simulink model "CM680A_HwTq2Meas"  (R2013b)
settings: Solver=FixedStepDiscrete  SolverMode=SingleTasking  StartTime=0.0  StopTime=1  FixedStep=0.002  RelTol=1e-3
values from neighbouring files (symbols this model uses):
  ELECGLBPRM_HWTQOFFS_HWNWTMTR_F32 = DataDict.Constant    [CM680A_HwTq2Meas_DataDict.m]
  ELECGLBPRM_HWTQSATNLOWRLIM_HWNWTMTR_F32 = DataDict.Constant    [CM680A_HwTq2Meas_DataDict.m]
  ELECGLBPRM_HWTQSATNUPPRLIM_HWNWTMTR_F32 = DataDict.Constant    [CM680A_HwTq2Meas_DataDict.m]
  ELECGLBPRM_HWTQSCA_ULS_F32 = DataDict.Constant    [CM680A_HwTq2Meas_DataDict.m]
  ELECGLBPRM_NOFLT_CNT_U08 = DataDict.Constant    [CM680A_HwTq2Meas_DataDict.m]
  ELECGLBPRM_OFFSTRIMNOTPRFM_CNT_U08 = DataDict.Constant    [CM680A_HwTq2Meas_DataDict.m]
  ELECGLBPRM_PRTCLFLT_CNT_U08 = DataDict.Constant    [CM680A_HwTq2Meas_DataDict.m]
  ELECGLBPRM_SNSRINTFLT_CNT_U08 = DataDict.Constant    [CM680A_HwTq2Meas_DataDict.m]
  FLTINJ_HWTQ2MEAS_HWTQ2 = DataDict.Constant    [CM680A_HwTq2Meas_DataDict.m]
  GearIdn1 = DataDict.OpSignal    [CM680A_HwTq2Meas_DataDict.m]
  HwTq2MeasHwTq2PrtclFltFailStep = DataDict.Calibration    [CM680A_HwTq2Meas_DataDict.m]
  HwTq2MeasHwTq2PrtclFltPassStep = DataDict.Calibration    [CM680A_HwTq2Meas_DataDict.m]
undefined symbols (not defined in the file or in its folder): NtcNr1, NtcSts1, sigbuilder_block, SigQlfr1
libraries: simulink x22, NxtrNvM x3
(part 3 of 3)

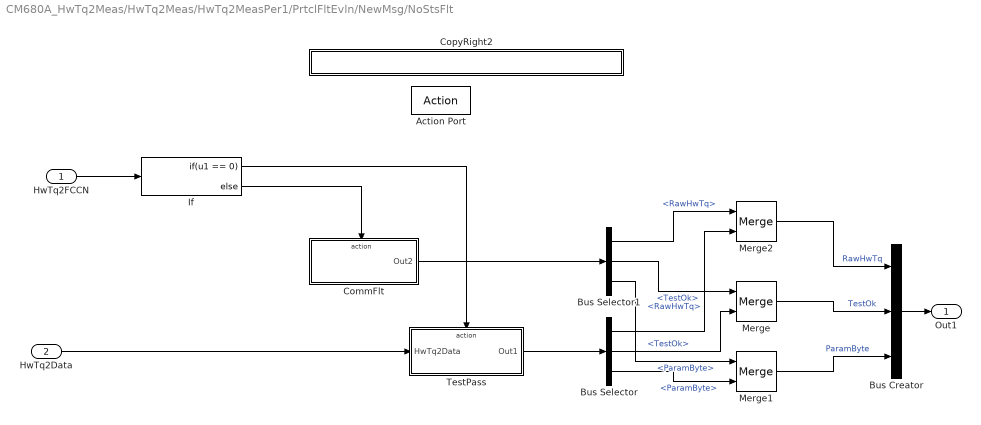
== system CM680A_HwTq2Meas/HwTq2Meas/HwTq2MeasPer1/PrtclFltEvln/NewMsg/NoStsFlt ==
  HwTq2FCCN : Inport
  HwTq2Data : Inport  Port=2
  Action Port : ActionPort  ActionType=then
  Bus Creator : BusCreator  Inputs=3
  Bus Selector : BusSelector  OutputSignals=RawHwTq,TestOk,ParamByte
  Bus Selector1 : BusSelector  OutputSignals=RawHwTq,TestOk,ParamByte
  CommFlt : Subsystem  RequirementInfo={'linktype_rmi_doors' '0000cf42 (/ESG Group/FDD Module Requirements/EA4 Specific/CM680A_HwTq2Meas)' '#CM680A_28' 'true' 'REQ: CM680A_28' '' ; 'linktype_rmi_doors' '0000cf42 (/ESG Group/FDD Module Requirements/EA4 Specific/CM680A_HwTq2Meas)' '#CM680A_48' 'true' 'REQ: CM680A_48' '' } %GIDa_a181911d_9433_49e5_ad17_4bc594fa1b0c  TreatAsAtomicUnit=on
      mask Display: disp('CommFlt')
  CopyRight2 : Subsystem  Description=|  mask(Copyright Information){none=on}
      | Copyright info block.                                               
      |                                                                     
      | Place copyright information at the top of every subsystem in design.
      mask prompts: none "No parameters"
      mask help: Place copyright information at the top of every subsystem in design.
      mask Display:
      | NxtrConf = 'Nexteer Confidential';
      | 
      | sys = bdroot; %handle for the current model ("system")
      | first = get_param(sys,'Created');
      | first = first(end-3:end);  %year is last four digits
      | 
      | last = get_param(sys,'LastModifiedDate');
      | if isempty(last)
      |     last = datestr(now,'yyyy');
      | else
      |     last = last(end-3:end);
      | end
      | 
      | if strcmp(first,last)
      |     fprintf('%s -- Copyright %s Nexteer',NxtrConf,first)
      | else
      |     fprintf('%s -- %s%s- %s Nexteer',NxtrConf,char(169),first,last)
      | end
  If : If  IfExpression=u1 == 0
  Merge : Merge
  Merge1 : Merge
  Merge2 : Merge
  TestPass : Subsystem  RequirementInfo={'linktype_rmi_doors' '0000cf42 (/ESG Group/FDD Module Requirements/EA4 Specific/CM680A_HwTq2Meas)' '#CM680A_49' 'true' 'REQ: CM680A_49' '' } %GIDa_eb2d61f5_a171_4ae7_8550_49e90430938b  TreatAsAtomicUnit=on
      mask Display: disp('TESTPASS')
  Out1 : Outport
  wires:
  HwTq2FCCN/1 -> If/1
  If/1 -> TestPass/Action
  If/2 -> CommFlt/Action
  Merge/1 -> Bus Creator/2  "TestOk"
  Merge1/1 -> Bus Creator/3  "ParamByte"
  Merge2/1 -> Bus Creator/1  "RawHwTq"
  TestPass/1(Out1) -> Bus Selector/1
  CommFlt/1(Out2) -> Bus Selector1/1
  Bus Selector1/1 -> Merge2/1  "<RawHwTq>"
  Bus Selector/1 -> Merge2/2  "<RawHwTq>"
  Bus Selector1/2 -> Merge/1  "<TestOk>"
  Bus Selector1/3 -> Merge1/1  "<ParamByte>"
  Bus Selector/2 -> Merge/2  "<TestOk>"
  Bus Selector/3 -> Merge1/2  "<ParamByte>"
  Bus Creator/1 -> Out1/1
  HwTq2Data/1 -> TestPass/1(HwTq2Data)

== system CM680A_HwTq2Meas/HwTq2Meas/HwTq2MeasPer1/PrtclFltEvln/NewMsg/StsFlt ==
  Action Port : ActionPort  ActionType=else
  Add : Sum
  Bus Creator : BusCreator  Inputs=3
  Constant : Constant  OutDataTypeStr=uint8
  CopyRight2 : Subsystem  Description=|  mask(Copyright Information){none=on}
      | Copyright info block.                                               
      |                                                                     
      | Place copyright information at the top of every subsystem in design.
      mask prompts: none "No parameters"
      mask help: Place copyright information at the top of every subsystem in design.
      mask Display:
      | NxtrConf = 'Nexteer Confidential';
      | 
      | sys = bdroot; %handle for the current model ("system")
      | first = get_param(sys,'Created');
      | first = first(end-3:end);  %year is last four digits
      | 
      | last = get_param(sys,'LastModifiedDate');
      | if isempty(last)
      |     last = datestr(now,'yyyy');
      | else
      |     last = last(end-3:end);
      | end
      | 
      | if strcmp(first,last)
      |     fprintf('%s -- Copyright %s Nexteer',NxtrConf,first)
      | else
      |     fprintf('%s -- %s%s- %s Nexteer',NxtrConf,char(169),first,last)
      | end
  Data Store Read : DataStoreRead  DataStoreName=HwTq2ComStsErrCntr
  Data Store Write : DataStoreWrite  DataStoreName=HwTq2ComStsErrCntr
  Data Type Conversion : DataTypeConversion  OutDataTypeStr=uint8
  HwTq : Constant  Value=0  OutDataTypeStr=uint32
  NtcSts : simulink/Sources/Enumerated Constant  OutDataTypeStr=Enum: NtcSts1  Value=NtcSts1.NTCSTS_PREFAILD  SampleTime=inf
  PRTCL_FAULT : Constant  Value=ELECGLBPRM_PRTCLFLT_CNT_U08  OutDataTypeStr=uint8
  Signal Conversion : SignalConversion
  Out1 : Outport
  wires:
  PRTCL_FAULT/1 -> Bus Creator/3  "ParamByte"
  NtcSts/1 -> Data Type Conversion/1
  HwTq/1 -> Bus Creator/1  "RawHwTq"
  Bus Creator/1 -> Signal Conversion/1
  Signal Conversion/1 -> Out1/1
  Data Type Conversion/1 -> Bus Creator/2  "TestOk"
  Data Store Read/1 -> Add/1
  Constant/1 -> Add/2
  Add/1 -> Data Store Write/1

== system CM680A_HwTq2Meas/HwTq2Meas/HwTq2MeasPer1/PrtclFltEvln/NoNewMsg/CopyRight2 ==

== system CM680A_HwTq2Meas/HwTq2Meas/HwTq2MeasPer1/SlowSerlDataRead/SlowSerlRead0/CopyRight2 ==

== system CM680A_HwTq2Meas/HwTq2Meas/HwTq2MeasPer1/SlowSerlDataRead/SlowSerlRead0/SlowSerlRead1 ==
  SlowSerlMsgID : Inport
  SlowSerlMsgData : Inport  Port=2
  Action Port : ActionPort  ActionType=then
  CopyRight2 : Subsystem  Description=|  mask(Copyright Information){none=on}
      | Copyright info block.                                               
      |                                                                     
      | Place copyright information at the top of every subsystem in design.
      mask prompts: none "No parameters"
      mask help: Place copyright information at the top of every subsystem in design.
      mask Display:
      | NxtrConf = 'Nexteer Confidential';
      | 
      | sys = bdroot; %handle for the current model ("system")
      | first = get_param(sys,'Created');
      | first = first(end-3:end);  %year is last four digits
      | 
      | last = get_param(sys,'LastModifiedDate');
      | if isempty(last)
      |     last = datestr(now,'yyyy');
      | else
      |     last = last(end-3:end);
      | end
      | 
      | if strcmp(first,last)
      |     fprintf('%s -- Copyright %s Nexteer',NxtrConf,first)
      | else
      |     fprintf('%s -- %s%s- %s Nexteer',NxtrConf,char(169),first,last)
      | end
  If : If  IfExpression=(u1==2)  ShowElse=off
  SlowSerlRead2 : Subsystem  TreatAsAtomicUnit=on
  wires:
  If/1 -> SlowSerlRead2/Action  "True"
  SlowSerlMsgID/1 -> If/1
  SlowSerlMsgData/1 -> SlowSerlRead2/1(SlowSerlMsgData)

== system CM680A_HwTq2Meas/HwTq2Meas/HwTq2MeasPer1/PrtclFltEvln/NewMsg/NoStsFlt/CommFlt ==
  Action Port : ActionPort  ActionType=else
  Add : Sum
  Bus Creator1 : BusCreator  Inputs=3
  Constant : Constant  OutDataTypeStr=uint8
  CopyRight2 : Subsystem  Description=|  mask(Copyright Information){none=on}
      | Copyright info block.                                               
      |                                                                     
      | Place copyright information at the top of every subsystem in design.
      mask prompts: none "No parameters"
      mask help: Place copyright information at the top of every subsystem in design.
      mask Display:
      | NxtrConf = 'Nexteer Confidential';
      | 
      | sys = bdroot; %handle for the current model ("system")
      | first = get_param(sys,'Created');
      | first = first(end-3:end);  %year is last four digits
      | 
      | last = get_param(sys,'LastModifiedDate');
      | if isempty(last)
      |     last = datestr(now,'yyyy');
      | else
      |     last = last(end-3:end);
      | end
      | 
      | if strcmp(first,last)
      |     fprintf('%s -- Copyright %s Nexteer',NxtrConf,first)
      | else
      |     fprintf('%s -- %s%s- %s Nexteer',NxtrConf,char(169),first,last)
      | end
  Data Store Read : DataStoreRead  DataStoreName=HwTq2IntSnsrErrCntr
  Data Store Write : DataStoreWrite  DataStoreName=HwTq2IntSnsrErrCntr
  Data Type Conversion : DataTypeConversion  OutDataTypeStr=uint8
  Flt : Constant  Value=ELECGLBPRM_SNSRINTFLT_CNT_U08  OutDataTypeStr=uint8
  HwTq : Constant  Value=0  OutDataTypeStr=uint32
  NtcSts : simulink/Sources/Enumerated Constant  OutDataTypeStr=Enum: NtcSts1  Value=NtcSts1.NTCSTS_PREFAILD  SampleTime=inf
  Signal Conversion1 : SignalConversion
  Out2 : Outport
  wires:
  Flt/1 -> Bus Creator1/3  "ParamByte"
  NtcSts/1 -> Data Type Conversion/1
  HwTq/1 -> Bus Creator1/1  "RawHwTq"
  Bus Creator1/1 -> Signal Conversion1/1
  Signal Conversion1/1 -> Out2/1
  Data Type Conversion/1 -> Bus Creator1/2  "TestOk"
  Data Store Read/1 -> Add/1
  Constant/1 -> Add/2
  Add/1 -> Data Store Write/1

== system CM680A_HwTq2Meas/HwTq2Meas/HwTq2MeasPer1/PrtclFltEvln/NewMsg/NoStsFlt/CopyRight2 ==

== system CM680A_HwTq2Meas/HwTq2Meas/HwTq2MeasPer1/PrtclFltEvln/NewMsg/NoStsFlt/TestPass ==
  HwTq2Data : Inport
  Action Port : ActionPort  ActionType=then
  Bus Creator : BusCreator  Inputs=3
  CopyRight2 : Subsystem  Description=|  mask(Copyright Information){none=on}
      | Copyright info block.                                               
      |                                                                     
      | Place copyright information at the top of every subsystem in design.
      mask prompts: none "No parameters"
      mask help: Place copyright information at the top of every subsystem in design.
      mask Display:
      | NxtrConf = 'Nexteer Confidential';
      | 
      | sys = bdroot; %handle for the current model ("system")
      | first = get_param(sys,'Created');
      | first = first(end-3:end);  %year is last four digits
      | 
      | last = get_param(sys,'LastModifiedDate');
      | if isempty(last)
      |     last = datestr(now,'yyyy');
      | else
      |     last = last(end-3:end);
      | end
      | 
      | if strcmp(first,last)
      |     fprintf('%s -- Copyright %s Nexteer',NxtrConf,first)
      | else
      |     fprintf('%s -- %s%s- %s Nexteer',NxtrConf,char(169),first,last)
      | end
  Data Type Conversion : DataTypeConversion  OutDataTypeStr=uint8
  NoFlt : Constant  RequirementInfo={} %GIDa_e64df96d_f0ef_4edd_b9a4_9c46566b9362  Value=ELECGLBPRM_NOFLT_CNT_U08  OutDataTypeStr=uint8
  NtcSts1 : simulink/Sources/Enumerated Constant  OutDataTypeStr=Enum: NtcSts1  Value=NtcSts1.NTCSTS_PREPASSD  SampleTime=inf
  Signal Conversion : SignalConversion
  Out1 : Outport
  wires:
  NtcSts1/1 -> Data Type Conversion/1
  Data Type Conversion/1 -> Bus Creator/2  "TestOk"
  NoFlt/1 -> Bus Creator/3  "ParamByte"
  HwTq2Data/1 -> Bus Creator/1  "RawHwTq"
  Bus Creator/1 -> Signal Conversion/1
  Signal Conversion/1 -> Out1/1

== system CM680A_HwTq2Meas/HwTq2Meas/HwTq2MeasPer1/PrtclFltEvln/NewMsg/StsFlt/CopyRight2 ==

== system CM680A_HwTq2Meas/HwTq2Meas/HwTq2MeasPer1/SlowSerlDataRead/SlowSerlRead0/SlowSerlRead1/CopyRight2 ==

== system CM680A_HwTq2Meas/HwTq2Meas/HwTq2MeasPer1/SlowSerlDataRead/SlowSerlRead0/SlowSerlRead1/SlowSerlRead2 ==
  SlowSerlMsgData : Inport
  Action Port : ActionPort  ActionType=then
  Constant : Constant  Value=true  OutDataTypeStr=boolean
      settings: AttributesFormatString=%<OutDataTypeStr>
  CopyRight2 : Subsystem  Description=|  mask(Copyright Information){none=on}
      | Copyright info block.                                               
      |                                                                     
      | Place copyright information at the top of every subsystem in design.
      mask prompts: none "No parameters"
      mask help: Place copyright information at the top of every subsystem in design.
      mask Display:
      | NxtrConf = 'Nexteer Confidential';
      | 
      | sys = bdroot; %handle for the current model ("system")
      | first = get_param(sys,'Created');
      | first = first(end-3:end);  %year is last four digits
      | 
      | last = get_param(sys,'LastModifiedDate');
      | if isempty(last)
      |     last = datestr(now,'yyyy');
      | else
      |     last = last(end-3:end);
      | end
      | 
      | if strcmp(first,last)
      |     fprintf('%s -- Copyright %s Nexteer',NxtrConf,first)
      | else
      |     fprintf('%s -- %s%s- %s Nexteer',NxtrConf,char(169),first,last)
      | end
  Data1 : DataStoreWrite  DataStoreName=GearIdn1Avl
  Data2 : DataStoreWrite  DataStoreName=GearIdn1Data
  wires:
  Constant/1 -> Data1/1
  SlowSerlMsgData/1 -> Data2/1

== system CM680A_HwTq2Meas/HwTq2Meas/HwTq2MeasPer1/PrtclFltEvln/NewMsg/NoStsFlt/CommFlt/CopyRight2 ==

== system CM680A_HwTq2Meas/HwTq2Meas/HwTq2MeasPer1/PrtclFltEvln/NewMsg/NoStsFlt/TestPass/CopyRight2 ==

== system CM680A_HwTq2Meas/HwTq2Meas/HwTq2MeasPer1/SlowSerlDataRead/SlowSerlRead0/SlowSerlRead1/SlowSerlRead2/CopyRight2 ==

== stateflow chart CM680A_HwTq2Meas/HwTq2Meas/HwTq2MeasPer2/SetNtcSts/ISO Fault Debounce Design ==
  settings: stateMachineType=MEALY_MACHINE
  note: NTCSTS_PASSD           (0)
      | NTCSTS_FAILD             (1)
      | NTCSTS_PREPASSD   (2)
      | NTCSTS_PREFAILD     (3)
      |
      | SIGQLFR_NORES        (0)
      | SIGQLFR_PASSD         (1)
      | SIGQLFR_FAILD           (2)
  note: Pass Loop
  note: Fail Loop
  note: 
  (default) -> (junction 89)
  (junction 89) -> (junction 95) [order 1] : [NtcSts ==3]
  (junction 89) -> (junction 93) [order 2] : [NtcSts ==2]
  (junction 89) -> (junction 141) [order 3] : [NtcSts ==1]
      | { ErrAcc = 32767;
      | Qualifier =2;
      |  }
  (junction 89) -> (junction 141) [order 4] : [NtcSts ==0]
      | { ErrAcc = -32768;
      | Qualifier=1;
      | }
  (junction 95) -> (junction 103) [order 2]
  (junction 95) -> (junction 111) [order 1] : [ErrAcc <=0]
      | {ErrAcc = DebStep;}
  (junction 93) -> (junction 123) [order 2] : {
      | ErrAcc = ErrAcc - DebStep;
      | }
  (junction 93) -> (junction 123) [order 1] : [(ErrAcc - DebStep) <= -32768]
      | { ErrAcc = -32768;
      | Qualifier=1;
      | }
  (junction 103) -> (junction 111) [order 1] : [(ErrAcc + DebStep) <32767]
      | {ErrAcc = ErrAcc + DebStep;}
  (junction 103) -> (junction 111) [order 2] : {ErrAcc = 32767;
      | Qualifier =2;}
  (junction 123) -> (junction 141)
  (junction 111) -> (junction 141)
  (junction 141) -> (junction 159) [order 2] : {ErrAcc = 0;
      | Qualifier =0;
      | }
  (junction 141) -> (junction 159) [order 1] : [SvcClr ==0]
  data: NtcSts input uint8; Qualifier output uint8; DebStep input uint16; ErrAcc local single; SvcClr input

== stateflow chart CM680A_HwTq2Meas/HwTq2Meas/HwTq2MeasPer1/SetNtcSts/ISO Fault Debounce Design ==
  settings: stateMachineType=MEALY_MACHINE
  note: NTCSTS_PASSD           (0)
      | NTCSTS_FAILD             (1)
      | NTCSTS_PREPASSD   (2)
      | NTCSTS_PREFAILD     (3)
      |
      | SIGQLFR_NORES        (0)
      | SIGQLFR_PASSD         (1)
      | SIGQLFR_FAILD           (2)
  note: Pass Loop
  note: Fail Loop
  note: 
  (default) -> (junction 89)
  (junction 89) -> (junction 95) [order 1] : [NtcSts ==3]
  (junction 89) -> (junction 93) [order 2] : [NtcSts ==2]
  (junction 89) -> (junction 141) [order 3] : [NtcSts ==1]
      | { ErrAcc = 32767;
      | Qualifier =2;
      |  }
  (junction 89) -> (junction 141) [order 4] : [NtcSts ==0]
      | { ErrAcc = -32768;
      | Qualifier=1;
      | }
  (junction 95) -> (junction 103) [order 2]
  (junction 95) -> (junction 111) [order 1] : [ErrAcc <=0]
      | {ErrAcc = DebStep;}
  (junction 93) -> (junction 123) [order 2] : {
      | ErrAcc = ErrAcc - DebStep;
      | }
  (junction 93) -> (junction 123) [order 1] : [(ErrAcc - DebStep) <= -32768]
      | { ErrAcc = -32768;
      | Qualifier=1;
      | }
  (junction 103) -> (junction 111) [order 1] : [(ErrAcc + DebStep) <32767]
      | {ErrAcc = ErrAcc + DebStep;}
  (junction 103) -> (junction 111) [order 2] : {ErrAcc = 32767;
      | Qualifier =2;}
  (junction 123) -> (junction 141)
  (junction 111) -> (junction 141)
  (junction 141) -> (junction 159) [order 2] : {ErrAcc = 0;
      | Qualifier =0;
      | }
  (junction 141) -> (junction 159) [order 1] : [SvcClr ==0]
  data: NtcSts input uint8; Qualifier output uint8; DebStep input uint16; ErrAcc local int16; SvcClr input

== stateflow chart CM680A_HwTq2Meas/HwTq2Meas/HwTq2MeasPer1/RollCnt1 ==
  settings: stateMachineType=MEALY_MACHINE
  (default) -> (junction 89) : {HwTq2RollgCntr = HwTq2PrevRollgCntr;}
  (junction 89) -> (junction 169) [order 1] : [ (TestOk ==2) ]
  (junction 89) -> (junction 93) [order 2]
  (junction 169) -> (junction 93) [order 2] : {HwTq2RollgCntr = 0;}
  (junction 169) -> (junction 93) [order 1] : [(HwTq2RollgCntr+1) <= 255]
      | {HwTq2RollgCntr = HwTq2RollgCntr + 1;}
  (junction 93) -> (junction 188)
  data: TestOk input uint8; HwTq2PrevRollgCntr input; HwTq2RollgCntr output uint8
